simulink model "Exemplo_1"  (R2012b)
settings: Solver=ode23t  StartTime=0.0  StopTime=10  MaxStep=0.2  RelTol=1e-3
libraries: fl_lib x9, nesl_utility x4, elec_lib x3
settings Model: Creator=Daniel  LastModifiedBy=Daniel

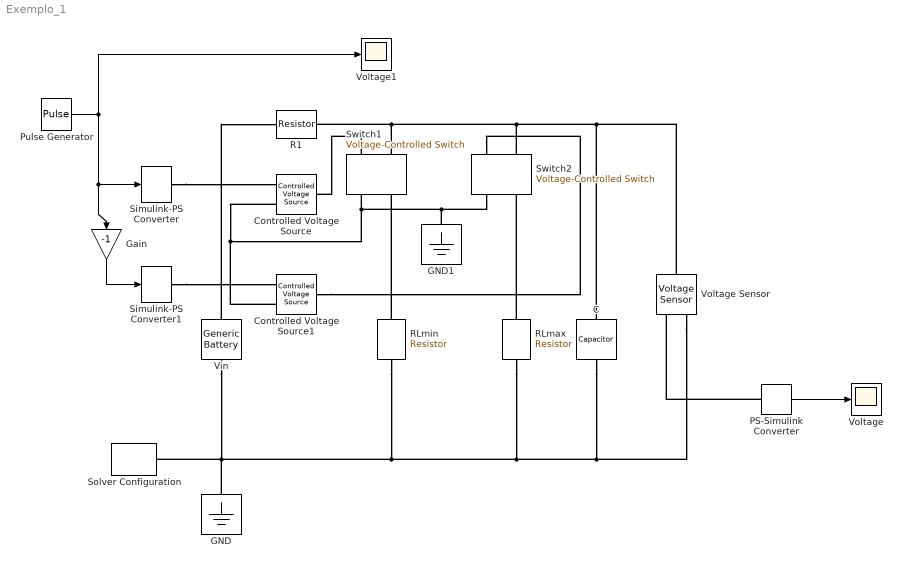
== system Exemplo_1 ==
  C : fl_lib/Electrical/Electrical Elements/Capacitor  c=100 uF  v0=2 V  r=1e-6 Ohm  g=0 1/Ohm  i_Log=off  v_Log=off  vc_Log=off  LocalVarNames=|i|v|vc  LocalVarDescs=|i|v|Internal variable for voltage across capacitor term  LocalVarLogging=[0 0 0]
  Controlled Voltage Source : fl_lib/Electrical/Electrical Sources/Controlled Voltage Source  i_Log=off  v_Log=off  LocalVarNames=|i|v  LocalVarDescs=|i|v  LocalVarLogging=[0 0]
  Controlled Voltage Source1 : fl_lib/Electrical/Electrical Sources/Controlled Voltage Source  i_Log=off  v_Log=off  LocalVarNames=|i|v  LocalVarDescs=|i|v  LocalVarLogging=[0 0]
  GND : fl_lib/Electrical/Electrical Elements/Electrical Reference  i_Log=off  LocalVarNames=|i  LocalVarDescs=|i  LocalVarLogging=0
  GND1 : fl_lib/Electrical/Electrical Elements/Electrical Reference  i_Log=off  LocalVarNames=|i  LocalVarDescs=|i  LocalVarLogging=0
  Gain : Gain  Gain=-1
  PS-Simulink Converter : nesl_utility/PS-Simulink Converter  PhysicalDomain=network_engine_domain  LeftPortType=input  RightPortType=output  SubClassName=ps_output  PseudoPeriodic=off  Frequencies=[]  Unit=1  AffineConversion=off
  Pulse Generator : DiscretePulseGenerator  PulseType=Time based  Amplitude=1.1  Period=1  PulseWidth=50
  R1 : fl_lib/Electrical/Electrical Elements/Resistor  R=15 Ohm  i_Log=off  v_Log=off  LocalVarNames=|i|v  LocalVarDescs=|i|v  LocalVarLogging=[0 0]
  RLmax : fl_lib/Electrical/Electrical Elements/Resistor  R=100 Ohm  i_Log=off  v_Log=off  LocalVarNames=|i|v  LocalVarDescs=|i|v  LocalVarLogging=[0 0]
  RLmin : fl_lib/Electrical/Electrical Elements/Resistor  R=10 Ohm  i_Log=off  v_Log=off  LocalVarNames=|i|v  LocalVarDescs=|i|v  LocalVarLogging=[0 0]
  Simulink-PS Converter : nesl_utility/Simulink-PS Converter  PhysicalDomain=network_engine_domain  LeftPortType=input  RightPortType=output  SubClassName=ps_input  PseudoPeriodic=off  Frequencies=[]  NoiseDistribution=none  NoiseParameters=[]  Unit=1  AffineConversion=off  InputFilterTimeConstant=.001  UdotUserProvided=[]  SimscapeFilterOrder=1  InputFiltering=off
  Simulink-PS Converter1 : nesl_utility/Simulink-PS Converter  PhysicalDomain=network_engine_domain  LeftPortType=input  RightPortType=output  SubClassName=ps_input  PseudoPeriodic=off  Frequencies=[]  NoiseDistribution=none  NoiseParameters=[]  Unit=1  AffineConversion=off  InputFilterTimeConstant=.001  UdotUserProvided=[]  SimscapeFilterOrder=1  InputFiltering=off
  Solver Configuration : nesl_utility/Solver Configuration  PhysicalDomain=network_engine_domain  LeftPortType=input  RightPortType=generic  SubClassName=solver  Accelerate=off  Profile=off  UseLocalSampling=off  FrequencyDomain=off  Tones=[]  Harmonics=[]  UseCCode=off  SimulateNoise=off  EnableSwitchedLinearOptims=on  DoDC=off  ResidualTolerance=1e-9  UseLocalSolver=off  LocalSolverChoice=NE_BACKWARD_EULER_ADVANCER  LocalSolverSampleTime=.001  DoFixedCost=off  MaxNonlinIter=3  MaxModeIter=2  LinearAlgebra=Sparse  DelaysMemoryBudget=1024
  Switch1 : elec_lib/Additional Components/SPICE-Compatible Components/Passive Devices/Voltage-Controlled Switch  VT=1 V  VH=0 V  RON=0.001 Ohm  ROFF=1e+12 Ohm  IC_state=1  LocalVarLogging=[]
  Switch2 : elec_lib/Additional Components/SPICE-Compatible Components/Passive Devices/Voltage-Controlled Switch  VT=1 V  VH=0 V  RON=0.001 Ohm  ROFF=1e+12 Ohm  IC_state=1  LocalVarLogging=[]
  Vin : elec_lib/Sources/Generic Battery  Vnom=5 V  R1=0.001 Ohm  prm_AH=1  AH=50 hr*A  AH0=50 hr*A  V1=11.5 V  AH1=25 hr*A  prm_R2=1  R2=2e+3 Ohm  LocalVarLogging=[]
  Voltage : Scope
  Voltage Sensor : fl_lib/Electrical/Electrical Sensors/Voltage Sensor  i1_Log=off  v1_Log=off  LocalVarNames=|i1|v1  LocalVarDescs=|i1|v1  LocalVarLogging=[0 0]
  Voltage1 : Scope
  wires:
  Pulse Generator/1 -> Simulink-PS Converter/1, Gain/1, Voltage1/1
  PS-Simulink Converter/1 -> Voltage/1
  Gain/1 -> Simulink-PS Converter1/1
  connections:
  GND/LConn1 -- RLmax/RConn1 -- Voltage Sensor/RConn2 -- C/RConn1 -- RLmin/RConn1 -- Vin/RConn1 -- Solver Configuration/RConn1
  R1/RConn1 -- Voltage Sensor/LConn1 -- C/LConn1 -- Switch2/LConn2 -- Switch1/LConn2
  Vin/LConn1 -- R1/LConn1
  PS-Simulink Converter/LConn1 -- Voltage Sensor/RConn1
  Simulink-PS Converter/RConn1 -- Controlled Voltage Source/RConn1
  RLmin/LConn1 -- Switch1/RConn2
  RLmax/LConn1 -- Switch2/RConn2
  Switch1/LConn1 -- Controlled Voltage Source/LConn1
  Switch2/RConn1 -- GND1/LConn1 -- Controlled Voltage Source1/RConn2 -- Controlled Voltage Source/RConn2 -- Switch1/RConn1
  Simulink-PS Converter1/RConn1 -- Controlled Voltage Source1/RConn1
  Controlled Voltage Source1/LConn1 -- Switch2/LConn1
